simulink model "InverterStartupControl"  (R2022b)
settings: Solver=FixedStepAuto  StartTime=0.0  StopTime=inf  FixedStep=0.005  RelTol=1e-3  EnableMultiTasking=on
undefined symbols (not defined in the file): MI_STATUSES, motor_interface, motor_interface_lib
libraries: simulink x1
settings Model: ExtModeTrigDuration=10  Creator=LinF  LastModifiedBy=LinF
settings SolverCC: AutoInsertRateTranBlk=on
settings OptimizationCC: EnhancedBackFolding=on  PassReuseOutputArgsAs=Individual arguments  ZeroExternalMemoryAtStartup=off  ZeroInternalMemoryAtStartup=off  MaxStackSize=64  OptimizeBlockOrder=speed  DifferentSizesBufferReuse=on  OptimizationCustomize=off  EfficientTunableParamExpr=on
settings DebuggingCC: ParameterTunabilityLossMsg=error
settings HardwareCC: ProdBitPerPointer=32  ProdBitPerSizeT=32  ProdBitPerPtrDiffT=32  ProdLargestAtomicInteger=Long  ProdLargestAtomicFloat=Double  ProdWordSize=32  ProdLongLongMode=on  ProdHWDeviceType=ARM Compatible->ARM Cortex  UseEmbeddedCoderFeatures=off
settings SFSimCC: MATLABDynamicMemAlloc=off
settings RTWCC: Description=Embedded Coder  SystemTargetFile=ert.tlc  HardwareBoard=STM32 Nucleo F767ZI  TLCOptions=-aInlineSetEventsForThisBaseRateFcn=TLC_FALSE -aSuppressMultiTaskScheduler=TLC_FALSE -aRateBasedStepFcn=1  GenCodeOnly=on  TemplateMakefile=ert_default_tmf  Toolchain=GNU Tools for ARM Embedded Processors
settings CodeAppCC: ForceParamTrailComments=on  IgnoreCustomStorageClasses=off  OperatorAnnotations=on  SimulinkDataObjDesc=on  SFDataObjDesc=on  InsertBlockDesc=on
settings ERTTargetCC: SupportNonInlinedSFcns=on  ExtModeTransport=3  ExtModeStaticAlloc=on  ExtModeStaticAllocSize=2000  ExtModeMexFile=ext_xcp  ExtModeIntrfLevel=Level2 - Open

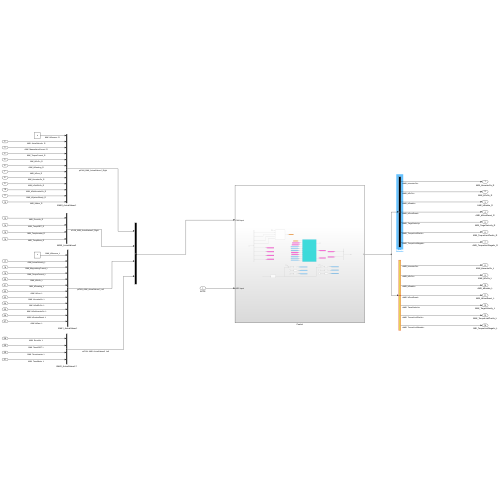
[thumbnail: Simulink's stored preview of the top-level diagram]
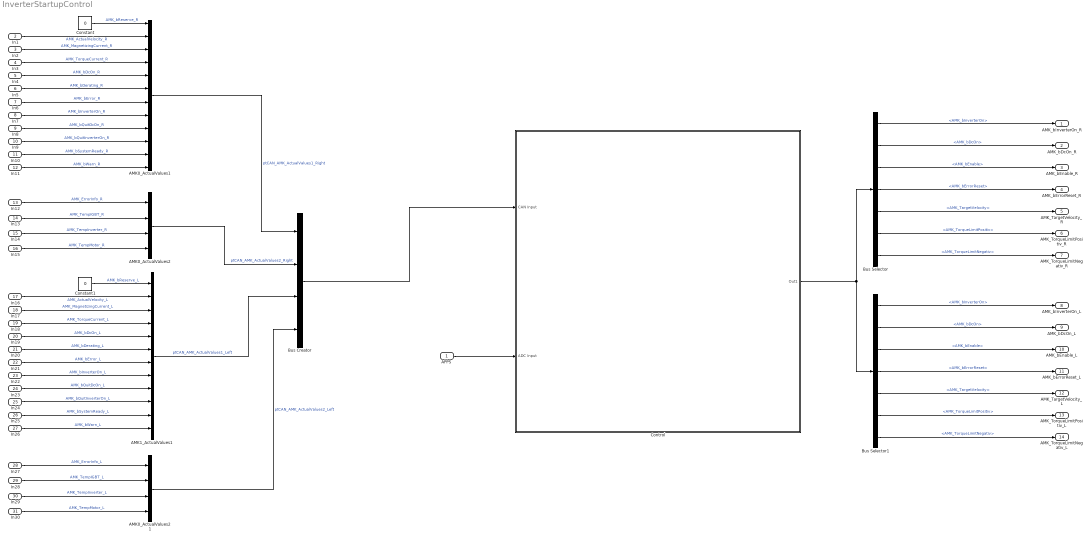
== system InverterStartupControl ==
  APPS : Inport
  In1 : Inport  Port=2
  In2 : Inport  Port=3
  In3 : Inport  Port=4
  In4 : Inport  Port=5
  In5 : Inport  Port=6
  In6 : Inport  Port=7
  In7 : Inport  Port=8
  In8 : Inport  Port=9
  In9 : Inport  Port=10
  In10 : Inport  Port=11
  In11 : Inport  Port=12
  In12 : Inport  Port=13
  In13 : Inport  Port=14
  In14 : Inport  Port=15
  In15 : Inport  Port=16
  In16 : Inport  Port=17
  In17 : Inport  Port=18
  In18 : Inport  Port=19
  In19 : Inport  Port=20
  In20 : Inport  Port=21
  In21 : Inport  Port=22
  In22 : Inport  Port=23
  In23 : Inport  Port=24
  In24 : Inport  Port=25
  In25 : Inport  Port=26
  In26 : Inport  Port=27
  In27 : Inport  Port=28
  In28 : Inport  Port=29
  In29 : Inport  Port=30
  In30 : Inport  Port=31
  "AMK0_ActualValues1 " : BusCreator  Inputs=12
  "AMK0_ActualValues2 " : BusCreator  Inputs=4
  AMK0_ActualValues2 1 : BusCreator  Inputs=4
  AMK1_ActualValues1 : BusCreator  Inputs=12
  Bus Creator : BusCreator  Inputs=4
  Bus Selector : BusSelector  OutputSignals=ptCAN_AMK_Setpoints1_Right.AMK_bInverterOn,ptCAN_AMK_Setpoints1_Right.AMK_bDcOn,ptCAN_AMK_Setpoints1_Right.AMK_bEnable,ptCAN_AMK_Setpoints1_Right.AMK_bErrorReset,ptCAN_AMK_Setpoints1_Right.AMK_TargetVelocity,ptCAN_AMK_Setpoints1_Right.AMK_TorqueLimitPositiv,ptCAN_AMK_Setpoints1_Right.AMK_TorqueLimitNegativ
  Bus Selector1 : BusSelector  OutputSignals=ptCAN_AMK_Setpoints1_Left.AMK_bInverterOn,ptCAN_AMK_Setpoints1_Left.AMK_bDcOn,ptCAN_AMK_Setpoints1_Left.AMK_bEnable,ptCAN_AMK_Setpoints1_Left.AMK_bErrorReset,ptCAN_AMK_Setpoints1_Left.AMK_TargetVelocity,ptCAN_AMK_Setpoints1_Left.AMK_TorqueLimitPositiv,ptCAN_AMK_Setpoints1_Left.AMK_TorqueLimitNegativ
  Constant : Constant  Value=0
  Constant1 : Constant  Value=0
  Control : Subsystem
  AMK_bInverterOn_R : Outport
  AMK_bDcOn_R : Outport  Port=2
  AMK_bEnable_R : Outport  Port=3
  AMK_bErrorReset_R : Outport  Port=4
  AMK_TargetVelocity_R : Outport  Port=5
  AMK_TorqueLimitPositiv_R : Outport  Port=6
  AMK_TorqueLimitNegativ_R : Outport  Port=7
  AMK_bInverterOn_L : Outport  Port=8
  AMK_bDcOn_L : Outport  Port=9
  AMK_bEnable_L : Outport  Port=10
  AMK_bErrorReset_L : Outport  Port=11
  AMK_TargetVelocity_L : Outport  Port=12
  AMK_TorqueLimitPositiv_L : Outport  Port=13
  AMK_TorqueLimitNegativ_L : Outport  Port=14
  wires:
  Bus Selector1/1 -> AMK_bInverterOn_L/1  "<AMK_bInverterOn>"
  Bus Selector/1 -> AMK_bInverterOn_R/1  "<AMK_bInverterOn>"
  Bus Selector1/7 -> AMK_TorqueLimitNegativ_L/1  "<AMK_TorqueLimitNegativ>"
  Bus Selector1/4 -> AMK_bErrorReset_L/1  "<AMK_bErrorReset>"
  Bus Selector1/3 -> AMK_bEnable_L/1  "<AMK_bEnable>"
  Bus Selector/5 -> AMK_TargetVelocity_R/1  "<AMK_TargetVelocity>"
  Bus Selector/4 -> AMK_bErrorReset_R/1  "<AMK_bErrorReset>"
  Bus Selector/3 -> AMK_bEnable_R/1  "<AMK_bEnable>"
  Bus Selector/7 -> AMK_TorqueLimitNegativ_R/1  "<AMK_TorqueLimitNegativ>"
  Bus Selector/6 -> AMK_TorqueLimitPositiv_R/1  "<AMK_TorqueLimitPositiv>"
  Bus Selector1/5 -> AMK_TargetVelocity_L/1  "<AMK_TargetVelocity>"
  Bus Selector1/6 -> AMK_TorqueLimitPositiv_L/1  "<AMK_TorqueLimitPositiv>"
  Bus Selector/2 -> AMK_bDcOn_R/1  "<AMK_bDcOn>"
  Control/1(Out1) -> Bus Selector/1, Bus Selector1/1
  Bus Selector1/2 -> AMK_bDcOn_L/1  "<AMK_bDcOn>"
  APPS/1 -> Control/2(ADC Input)
  In16/1 -> AMK1_ActualValues1/2  "AMK_ActualVelocity_L"
  In21/1 -> AMK1_ActualValues1/7  "AMK_bError_L"
  In11/1 -> "AMK0_ActualValues1 "/12  "AMK_bWarn_R"
  In10/1 -> "AMK0_ActualValues1 "/11  "AMK_bSystemReady_R"
  In28/1 -> AMK0_ActualValues2 1/2  "AMK_TempIGBT_L"
  In18/1 -> AMK1_ActualValues1/4  "AMK_TorqueCurrent_L"
  In4/1 -> "AMK0_ActualValues1 "/5  "AMK_bDcOn_R"
  In9/1 -> "AMK0_ActualValues1 "/10  "AMK_bQuitInverterOn_R"
  In25/1 -> AMK1_ActualValues1/11  "AMK_bSystemReady_L"
  In19/1 -> AMK1_ActualValues1/5  "AMK_bDcOn_L"
  In22/1 -> AMK1_ActualValues1/8  "AMK_bInverterOn_L"
  In12/1 -> "AMK0_ActualValues2 "/1  "AMK_ErrorInfo_R"
  In23/1 -> AMK1_ActualValues1/9  "AMK_bQuitDcOn_L"
  In30/1 -> AMK0_ActualValues2 1/4  "AMK_TempMotor_L"
  In6/1 -> "AMK0_ActualValues1 "/7  "AMK_bError_R"
  In27/1 -> AMK0_ActualValues2 1/1  "AMK_ErrorInfo_L"
  In17/1 -> AMK1_ActualValues1/3  "AMK_MagnetizingCurrent_L"
  In29/1 -> AMK0_ActualValues2 1/3  "AMK_TempInverter_L"
  In1/1 -> "AMK0_ActualValues1 "/2  "AMK_ActualVelocity_R"
  In5/1 -> "AMK0_ActualValues1 "/6  "AMK_bDerating_R"
  In24/1 -> AMK1_ActualValues1/10  "AMK_bQuitInverterOn_L"
  In20/1 -> AMK1_ActualValues1/6  "AMK_bDerating_L"
  In15/1 -> "AMK0_ActualValues2 "/4  "AMK_TempMotor_R"
  In14/1 -> "AMK0_ActualValues2 "/3  "AMK_TempInverter_R"
  AMK1_ActualValues1/1 -> Bus Creator/3  "ptCAN_AMK_ActualValues1_Left"
  In13/1 -> "AMK0_ActualValues2 "/2  "AMK_TempIGBT_R"
  Constant1/1 -> AMK1_ActualValues1/1  "AMK_bReserve_L"
  In8/1 -> "AMK0_ActualValues1 "/9  "AMK_bQuitDcOn_R"
  In3/1 -> "AMK0_ActualValues1 "/4  "AMK_TorqueCurrent_R"
  AMK0_ActualValues2 1/1 -> Bus Creator/4  "ptCAN_AMK_ActualValues2_Left"
  In2/1 -> "AMK0_ActualValues1 "/3  "AMK_MagnetizingCurrent_R"
  Bus Creator/1 -> Control/1(CAN Input)
  Constant/1 -> "AMK0_ActualValues1 "/1  "AMK_bReserve_R"
  "AMK0_ActualValues1 "/1 -> Bus Creator/1  "ptCAN_AMK_ActualValues1_Right"
  In7/1 -> "AMK0_ActualValues1 "/8  "AMK_bInverterOn_R"
  In26/1 -> AMK1_ActualValues1/12  "AMK_bWarn_L"
  "AMK0_ActualValues2 "/1 -> Bus Creator/2  "ptCAN_AMK_ActualValues2_Right"

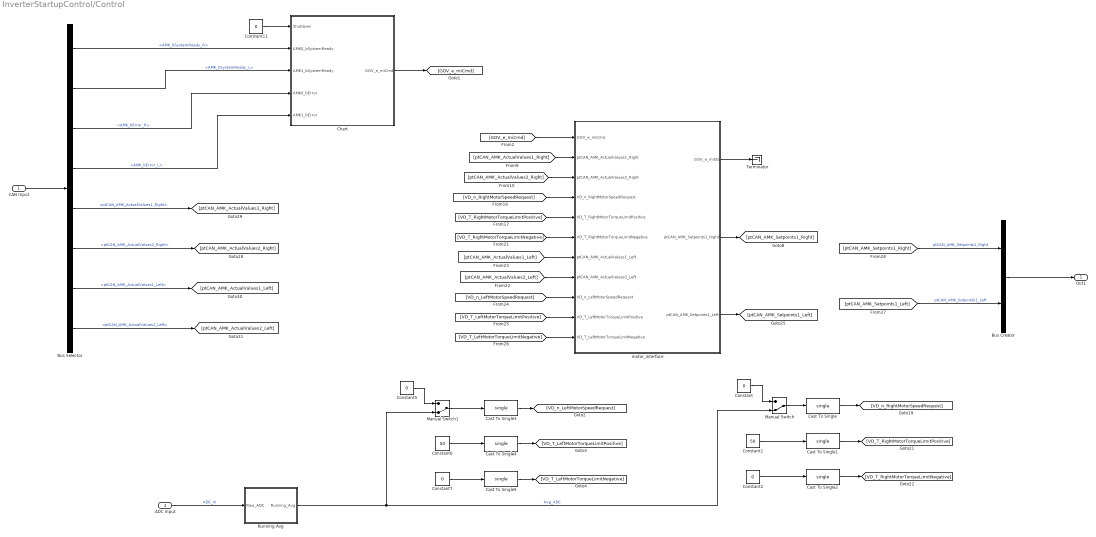
== system InverterStartupControl/Control ==
  CAN Input : Inport
  ADC Input : Inport  Port=2
  Bus Creator : BusCreator  Inputs=2
  Bus Selector : BusSelector  OutputSignals=ptCAN_AMK_ActualValues1_Right.AMK_bSystemReady_R,ptCAN_AMK_ActualValues1_Left.AMK_bSystemReady_L,ptCAN_AMK_ActualValues1_Right.AMK_bError_R,ptCAN_AMK_ActualValues1_Left.AMK_bError_L,ptCAN_AMK_ActualValues1_Right,ptCAN_AMK_ActualValues2_Right,ptCAN_AMK_ActualValues1_Left,ptCAN_AMK_ActualValues2_Left
  Cast To Single{,1..5} (6 alike) : DataTypeConversion  OutDataTypeStr=single  SaturateOnIntegerOverflow=off  RndMeth=Floor
  Chart : Stateflow chart  TreatAsAtomicUnit=on
  Constant{,2,5,7,11} (5 alike) : Constant  Value=0
  Constant1 : Constant  Value=50
  Constant6 : Constant  Value=50
  Manual Switch : ManualSwitch  CurrentSetting=0
  Manual Switch1 : ManualSwitch  CurrentSetting=0
  Running Avg : Subsystem
  Terminator : Terminator
  motor_interface : Subsystem  AncestorBlock=motor_interface_lib/motor_interface
      settings: LibrarySourceBlock=motor_interface_lib/motor_interface
  Out1 : Outport
  wires:
  [VD_T_RightMotorTorqueLimitPositive] -> motor_interface/5(VD_T_RightMotorTorqueLimitPositive)
  [ptCAN_AMK_ActualValues2_Right] -> motor_interface/3(ptCAN_AMK_ActualValues2_Right)
  [ptCAN_AMK_ActualValues2_Left] -> motor_interface/8(ptCAN_AMK_ActualValues2_Left)
  [VD_n_LeftMotorSpeedRequest] -> motor_interface/9(VD_n_LeftMotorSpeedRequest)
  [VD_T_LeftMotorTorqueLimitNegative] -> motor_interface/11(VD_T_LeftMotorTorqueLimitNegative)
  [VD_T_RightMotorTorqueLimitNegative] -> motor_interface/6(VD_T_RightMotorTorqueLimitNegative)
  motor_interface/2(ptCAN_AMK_Setpoints1_Right) -> [ptCAN_AMK_Setpoints1_Right]
  motor_interface/3(ptCAN_AMK_Setpoints1_Left) -> [ptCAN_AMK_Setpoints1_Left]
  [VD_T_LeftMotorTorqueLimitPositive] -> motor_interface/10(VD_T_LeftMotorTorqueLimitPositive)
  [VD_n_RightMotorSpeedRequest] -> motor_interface/4(VD_n_RightMotorSpeedRequest)
  [ptCAN_AMK_ActualValues1_Left] -> motor_interface/7(ptCAN_AMK_ActualValues1_Left)
  motor_interface/1(GOV_e_miSts) -> Terminator/1
  [GOV_e_miCmd] -> motor_interface/1(GOV_e_miCmd)
  [ptCAN_AMK_ActualValues1_Right] -> motor_interface/2(ptCAN_AMK_ActualValues1_Right)
  CAN Input/1 -> Bus Selector/1
  Bus Selector/6 -> [ptCAN_AMK_ActualValues2_Right]  "<ptCAN_AMK_ActualValues2_Right>"
  Constant2/1 -> Cast To Single2/1
  Bus Selector/8 -> [ptCAN_AMK_ActualValues2_Left]  "<ptCAN_AMK_ActualValues2_Left>"
  Constant7/1 -> Cast To Single5/1
  Manual Switch1/1 -> Cast To Single3/1
  Chart/1(GOV_e_miCmd) -> [GOV_e_miCmd]
  [ptCAN_AMK_Setpoints1_Right] -> Bus Creator/1  "ptCAN_AMK_Setpoints1_Right"
  [ptCAN_AMK_Setpoints1_Left] -> Bus Creator/2  "ptCAN_AMK_Setpoints1_Left"
  Bus Creator/1 -> Out1/1
  Bus Selector/5 -> [ptCAN_AMK_ActualValues1_Right]  "<ptCAN_AMK_ActualValues1_Right>"
  Bus Selector/1 -> Chart/2(AMK0_bSystemReady)  "<AMK_bSystemReady_R>"
  Bus Selector/3 -> Chart/4(AMK0_bError)  "<AMK_bError_R>"
  Constant/1 -> Manual Switch/1
  Manual Switch/1 -> Cast To Single/1
  Constant11/1 -> Chart/1(Shutdown)
  Bus Selector/7 -> [ptCAN_AMK_ActualValues1_Left]  "<ptCAN_AMK_ActualValues1_Left>"
  Cast To Single/1 -> [VD_n_RightMotorSpeedRequest]
  Cast To Single1/1 -> [VD_T_RightMotorTorqueLimitPositive]
  Cast To Single2/1 -> [VD_T_RightMotorTorqueLimitNegative]
  Cast To Single3/1 -> [VD_n_LeftMotorSpeedRequest]
  Cast To Single4/1 -> [VD_T_LeftMotorTorqueLimitPositive]
  Cast To Single5/1 -> [VD_T_LeftMotorTorqueLimitNegative]
  Bus Selector/2 -> Chart/3(AMK1_bSystemReady)  "<AMK_bSystemReady_L>"
  Bus Selector/4 -> Chart/5(AMK1_bError)  "<AMK_bError_L>"
  Constant5/1 -> Manual Switch1/1
  ADC Input/1 -> Running Avg/1(Raw_ADC)  "ADC_In"
  Running Avg/1(Running_Avg) -> Manual Switch/2, Manual Switch1/2  "Avg_ADC"
  Constant1/1 -> Cast To Single1/1
  Constant6/1 -> Cast To Single4/1

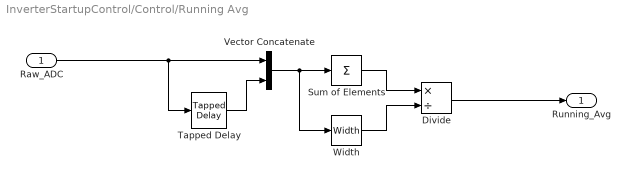
== system InverterStartupControl/Control/Running Avg ==
  Raw_ADC : Inport
  Divide : Product  Inputs=*/
  Sum of Elements : Sum  Inputs=+
  Tapped Delay : simulink/Discrete/Tapped Delay  vinit=0  samptime=-1  NumDelays=5  DelayOrder=Oldest  includeCurrent=off
  Vector Concatenate : Concatenate
  Width : Width
  Running_Avg : Outport
  wires:
  Divide/1 -> Running_Avg/1
  Vector Concatenate/1 -> Width/1, Sum of Elements/1
  Raw_ADC/1 -> Vector Concatenate/1, Tapped Delay/1
  Width/1 -> Divide/2
  Tapped Delay/1 -> Vector Concatenate/2
  Sum of Elements/1 -> Divide/1

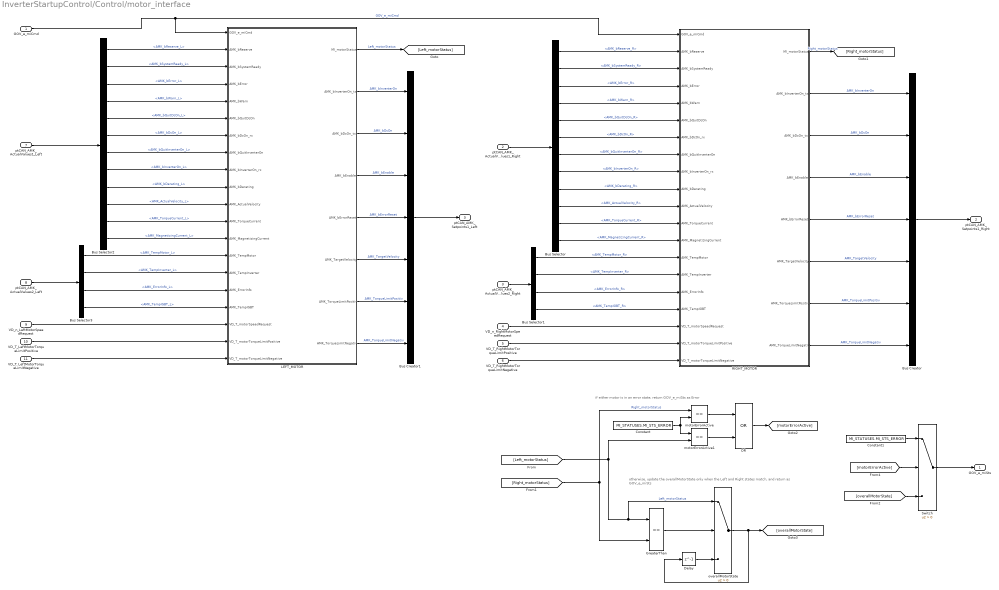
== system InverterStartupControl/Control/motor_interface ==
  note: otherwise, update the overallMotorState only when the Left and Right states match, and return as GOV_e_miSts
  note: if either motor is in an error state, return GOV_e_miSts as Error
  GOV_e_miCmd : Inport
  ptCAN_AMK_ActualValues1_Right : Inport  Port=2
  ptCAN_AMK_ActualValues2_Right : Inport  Port=3
  VD_n_RightMotorSpeedRequest : Inport  Port=4
  VD_T_RightMotorTorqueLimitPositive : Inport  Port=5
  VD_T_RightMotorTorqueLimitNegative : Inport  Port=6
  ptCAN_AMK_ActualValues1_Left : Inport  Port=7
  ptCAN_AMK_ActualValues2_Left : Inport  Port=8
  VD_n_LeftMotorSpeedRequest : Inport  Port=9
  VD_T_LeftMotorTorqueLimitPositive : Inport  Port=10
  VD_T_LeftMotorTorqueLimitNegative : Inport  Port=11
  Bus Creator : BusCreator  Inputs=7
  Bus Creator1 : BusCreator  Inputs=7
  Bus Selector : BusSelector  OutputSignals=AMK_bReserve_R,AMK_bSystemReady_R,AMK_bError_R,AMK_bWarn_R,AMK_bQuitDcOn_R,AMK_bDcOn_R,AMK_bQuitInverterOn_R,AMK_bInverterOn_R,AMK_bDerating_R,AMK_ActualVelocity_R,AMK_TorqueCurrent_R,AMK_MagnetizingCurrent_R
  Bus Selector1 : BusSelector  OutputSignals=AMK_TempMotor_R,AMK_TempInverter_R,AMK_ErrorInfo_R,AMK_TempIGBT_R
  Bus Selector2 : BusSelector  OutputSignals=AMK_bReserve_L,AMK_bSystemReady_L,AMK_bError_L,AMK_bWarn_L,AMK_bQuitDcOn_L,AMK_bDcOn_L,AMK_bQuitInverterOn_L,AMK_bInverterOn_L,AMK_bDerating_L,AMK_ActualVelocity_L,AMK_TorqueCurrent_L,AMK_MagnetizingCurrent_L
  Bus Selector3 : BusSelector  OutputSignals=AMK_TempMotor_L,AMK_TempInverter_L,AMK_ErrorInfo_L,AMK_TempIGBT_L
  Constant : Constant  Value=MI_STATUSES.MI_STS_ERROR  OutDataTypeStr=Enum: MI_STATUSES
  Constant1 : Constant  Value=MI_STATUSES.MI_STS_ERROR  OutDataTypeStr=Enum: MI_STATUSES
  Delay : Delay  DelayLength=1  InitialCondition=MI_STATUSES.OFF
  GreaterThan : RelationalOperator  Operator===  OutDataTypeStr=boolean  RndMeth=Simplest  InputSameDT=off
  LEFT_MOTOR : Stateflow chart  TreatAsAtomicUnit=on
  OR : Logic  Operator=OR  IconShape=distinctive  AllPortsSameDT=off  OutDataTypeStr=boolean
  RIGHT_MOTOR : Stateflow chart  TreatAsAtomicUnit=on
  Switch : Switch  Criteria=u2 > Threshold  SaturateOnIntegerOverflow=off  InputSameDT=off
  motorErrorActive : RelationalOperator  Operator===  OutDataTypeStr=boolean  RndMeth=Simplest  InputSameDT=off
  motorErrorActive1 : RelationalOperator  Operator===  OutDataTypeStr=boolean  RndMeth=Simplest  InputSameDT=off
  overallMotorState : Switch  Criteria=u2 > Threshold  SaturateOnIntegerOverflow=off  InputSameDT=off
  GOV_e_miSts : Outport
  ptCAN_AMK_Setpoints1_Right : Outport  Port=2
  ptCAN_AMK_Setpoints1_Left : Outport  Port=3
  wires:
  GOV_e_miCmd/1 -> LEFT_MOTOR/1(GOV_e_miCmd), RIGHT_MOTOR/1(GOV_e_miCmd)  "GOV_e_miCmd"
  ptCAN_AMK_ActualValues1_Right/1 -> Bus Selector/1
  Bus Selector/2 -> RIGHT_MOTOR/3(AMK_bSystemReady)  "<AMK_bSystemReady_R>"
  Bus Selector/3 -> RIGHT_MOTOR/4(AMK_bError)  "<AMK_bError_R>"
  Bus Selector/4 -> RIGHT_MOTOR/5(AMK_bWarn)  "<AMK_bWarn_R>"
  Bus Selector/5 -> RIGHT_MOTOR/6(AMK_bQuitDcOn)  "<AMK_bQuitDcOn_R>"
  Bus Selector/6 -> RIGHT_MOTOR/7(AMK_bDcOn_rx)  "<AMK_bDcOn_R>"
  Bus Selector/7 -> RIGHT_MOTOR/8(AMK_bQuitInverterOn)  "<AMK_bQuitInverterOn_R>"
  Bus Selector/8 -> RIGHT_MOTOR/9(AMK_bInverterOn_rx)  "<AMK_bInverterOn_R>"
  Bus Selector/9 -> RIGHT_MOTOR/10(AMK_bDerating)  "<AMK_bDerating_R>"
  Bus Selector/10 -> RIGHT_MOTOR/11(AMK_ActualVelocity)  "<AMK_ActualVelocity_R>"
  Bus Selector/11 -> RIGHT_MOTOR/12(AMK_TorqueCurrent)  "<AMK_TorqueCurrent_R>"
  Bus Selector/12 -> RIGHT_MOTOR/13(AMK_MagnetizingCurrent)  "<AMK_MagnetizingCurrent_R>"
  Bus Selector/1 -> RIGHT_MOTOR/2(AMK_bReserve)  "<AMK_bReserve_R>"
  ptCAN_AMK_ActualValues2_Right/1 -> Bus Selector1/1
  Bus Selector1/1 -> RIGHT_MOTOR/14(AMK_TempMotor)  "<AMK_TempMotor_R>"
  Bus Selector1/2 -> RIGHT_MOTOR/15(AMK_TempInverter)  "<AMK_TempInverter_R>"
  Bus Selector1/3 -> RIGHT_MOTOR/16(AMK_ErrorInfo)  "<AMK_ErrorInfo_R>"
  Bus Selector1/4 -> RIGHT_MOTOR/17(AMK_TempIGBT)  "<AMK_TempIGBT_R>"
  Bus Creator/1 -> ptCAN_AMK_Setpoints1_Right/1
  RIGHT_MOTOR/2(AMK_bInverterOn_tx) -> Bus Creator/1  "AMK_bInverterOn"
  RIGHT_MOTOR/4(AMK_bEnable) -> Bus Creator/3  "AMK_bEnable"
  RIGHT_MOTOR/6(AMK_TargetVelocity) -> Bus Creator/5  "AMK_TargetVelocity"
  RIGHT_MOTOR/3(AMK_bDcOn_tx) -> Bus Creator/2  "AMK_bDcOn"
  RIGHT_MOTOR/5(AMK_bErrorReset) -> Bus Creator/4  "AMK_bErrorReset"
  LEFT_MOTOR/1(MI_motorStatus) -> [Left_motorStatus]  "Left_motorStatus"
  RIGHT_MOTOR/1(MI_motorStatus) -> [Right_motorStatus]  "Right_motorStatus"
  [Left_motorStatus] -> motorErrorActive1/2, overallMotorState/1, GreaterThan/1  "Left_motorStatus"
  [Right_motorStatus] -> motorErrorActive/1, GreaterThan/2  "Right_motorStatus"
  Constant/1 -> motorErrorActive/2, motorErrorActive1/1
  Switch/1 -> GOV_e_miSts/1
  [motorErrorActive] -> Switch/2
  overallMotorState/1 -> Delay/1, [overallMotorState]
  Delay/1 -> overallMotorState/3
  GreaterThan/1 -> overallMotorState/2
  [overallMotorState] -> Switch/3
  OR/1 -> [motorErrorActive]
  motorErrorActive1/1 -> OR/2
  motorErrorActive/1 -> OR/1
  Constant1/1 -> Switch/1
  RIGHT_MOTOR/7(AMK_TorqueLimitPositiv) -> Bus Creator/6  "AMK_TorqueLimitPositiv"
  RIGHT_MOTOR/8(AMK_TorqueLimitNegativ) -> Bus Creator/7  "AMK_TorqueLimitNegativ"
  VD_T_RightMotorTorqueLimitPositive/1 -> RIGHT_MOTOR/19(VD_T_motorTorqueLimitPositive)
  VD_T_RightMotorTorqueLimitNegative/1 -> RIGHT_MOTOR/20(VD_T_motorTorqueLimitNegative)
  VD_n_RightMotorSpeedRequest/1 -> RIGHT_MOTOR/18(VD_T_motorSpeedRequest)
  VD_n_LeftMotorSpeedRequest/1 -> LEFT_MOTOR/18(VD_T_motorSpeedRequest)
  VD_T_LeftMotorTorqueLimitNegative/1 -> LEFT_MOTOR/20(VD_T_motorTorqueLimitNegative)
  VD_T_LeftMotorTorqueLimitPositive/1 -> LEFT_MOTOR/19(VD_T_motorTorqueLimitPositive)
  Bus Selector3/4 -> LEFT_MOTOR/17(AMK_TempIGBT)  "<AMK_TempIGBT_L>"
  Bus Selector3/3 -> LEFT_MOTOR/16(AMK_ErrorInfo)  "<AMK_ErrorInfo_L>"
  Bus Selector3/2 -> LEFT_MOTOR/15(AMK_TempInverter)  "<AMK_TempInverter_L>"
  Bus Selector3/1 -> LEFT_MOTOR/14(AMK_TempMotor)  "<AMK_TempMotor_L>"
  Bus Selector2/1 -> LEFT_MOTOR/2(AMK_bReserve)  "<AMK_bReserve_L>"
  Bus Selector2/12 -> LEFT_MOTOR/13(AMK_MagnetizingCurrent)  "<AMK_MagnetizingCurrent_L>"
  Bus Selector2/11 -> LEFT_MOTOR/12(AMK_TorqueCurrent)  "<AMK_TorqueCurrent_L>"
  Bus Selector2/10 -> LEFT_MOTOR/11(AMK_ActualVelocity)  "<AMK_ActualVelocity_L>"
  Bus Selector2/9 -> LEFT_MOTOR/10(AMK_bDerating)  "<AMK_bDerating_L>"
  Bus Selector2/8 -> LEFT_MOTOR/9(AMK_bInverterOn_rx)  "<AMK_bInverterOn_L>"
  Bus Selector2/7 -> LEFT_MOTOR/8(AMK_bQuitInverterOn)  "<AMK_bQuitInverterOn_L>"
  Bus Selector2/6 -> LEFT_MOTOR/7(AMK_bDcOn_rx)  "<AMK_bDcOn_L>"
  Bus Selector2/5 -> LEFT_MOTOR/6(AMK_bQuitDcOn)  "<AMK_bQuitDcOn_L>"
  Bus Selector2/4 -> LEFT_MOTOR/5(AMK_bWarn)  "<AMK_bWarn_L>"
  Bus Selector2/3 -> LEFT_MOTOR/4(AMK_bError)  "<AMK_bError_L>"
  Bus Selector2/2 -> LEFT_MOTOR/3(AMK_bSystemReady)  "<AMK_bSystemReady_L>"
  ptCAN_AMK_ActualValues1_Left/1 -> Bus Selector2/1
  LEFT_MOTOR/8(AMK_TorqueLimitNegativ) -> Bus Creator1/7  "AMK_TorqueLimitNegativ"
  LEFT_MOTOR/7(AMK_TorqueLimitPositiv) -> Bus Creator1/6  "AMK_TorqueLimitPositiv"
  LEFT_MOTOR/5(AMK_bErrorReset) -> Bus Creator1/4  "AMK_bErrorReset"
  LEFT_MOTOR/3(AMK_bDcOn_tx) -> Bus Creator1/2  "AMK_bDcOn"
  LEFT_MOTOR/6(AMK_TargetVelocity) -> Bus Creator1/5  "AMK_TargetVelocity"
  LEFT_MOTOR/4(AMK_bEnable) -> Bus Creator1/3  "AMK_bEnable"
  LEFT_MOTOR/2(AMK_bInverterOn_tx) -> Bus Creator1/1  "AMK_bInverterOn"
  Bus Creator1/1 -> ptCAN_AMK_Setpoints1_Left/1
  ptCAN_AMK_ActualValues2_Left/1 -> Bus Selector3/1

== stateflow chart InverterStartupControl/Control/Chart ==
  state Init
    en:
    GOV_e_miCmd = MI_CMD.CMD_INIT;
  state Run
    en:
    GOV_e_miCmd = MI_CMD.CMD_STARTUP;
  state Error0
    en:
    GOV_e_miCmd = MI_CMD.ERR_RESET;
  state Error1
    en:
    GOV_e_miCmd = MI_CMD.ERR_RESET;
  state Shutdown
    en:
    GOV_e_miCmd = MI_CMD.CMD_SHUTDOWN;
  (default) -> Init
  Shutdown -> Init : [Shutdown == 0]
  Init -> Run : [(AMK0_bSystemReady == 1 && AMK1_bSystemReady == 1) && Shutdown == 0]
  Run -> Error0 [order 1] : [AMK0_bError == 1]
  Error0 -> Run : [AMK0_bError == 0]
  Run -> Error1 [order 3] : [AMK1_bError == 1]
  Error1 -> Run : [AMK1_bError == 0]
  Run -> Shutdown [order 2] : [Shutdown == 1]
  data: Shutdown input; GOV_e_miCmd output; AMK0_bSystemReady input; AMK1_bSystemReady input; AMK0_bError input; AMK1_bError input

== stateflow chart InverterStartupControl/Control/motor_interface/LEFT_MOTOR ==
  note: [AMK_bError==1]
  state motorOff_waitingForGov
    en:
    MI_motorStatus = MI_STATUSES.OFF;
    AMK_bInverterOn_tx = 0;
    AMK_bDcOn_tx = 0;
    AMK_bEnable = 0;
    AMK_bErrorReset = 0;
    AMK_TargetVelocity = 0;
    AMK_TorqueLimitPositiv = 0;
    AMK_TorqueLimitNegativ = 0;
  state AMK_startup
    state waiting_sysReady
      en:
      MI_motorStatus = MI_STATUSES.STARTUP;
    state toggleDCon
      en:
      AMK_bDcOn_tx = 1;
    state enforceSetpointsZero
      en:
      AMK_TargetVelocity = 0;
      AMK_TorqueLimitPositiv = 0;
      AMK_TorqueLimitNegativ = 0;
    state commandOn
      en:
      AMK_bEnable = 1;
      AMK_bInverterOn_tx = 1;
    waiting_sysReady -> (junction 67) [order 2] : [AMK_bError==1]
    waiting_sysReady -> AMK_startup.toggleDCon [order 1] : [AMK_bSystemReady==1]
    AMK_startup.toggleDCon -> (junction 67) [order 2] : [AMK_bError==1]
    AMK_startup.toggleDCon -> AMK_startup.enforceSetpointsZero [order 1] : [(AMK_bDcOn_rx==1) ...
        | && (AMK_bQuitDcOn==1)]
    AMK_startup.enforceSetpointsZero -> (junction 67) [order 2] : [AMK_bError==1]
    commandOn -> (junction 67) [order 2] : [AMK_bError==1]
    AMK_startup.enforceSetpointsZero -> commandOn [order 1] : after(1,sec)
  state AMK_errorReset
    state toggleReset
      en:
      AMK_bErrorReset = 0;
    state sendReset
      en:
      AMK_bErrorReset = 1;
    state toggleEnable
      en:
      AMK_bEnable = 0;
    state enforceSetpointsZero
      en:
      AMK_TargetVelocity = 0;
      AMK_TorqueLimitPositiv = 0;
      AMK_TorqueLimitNegativ = 0;
      AMK_bInverterOn_tx = 0;
    sendReset -> toggleReset : after(500,msec)
    toggleEnable -> sendReset : after(500,msec)
    AMK_errorReset.enforceSetpointsZero -> toggleEnable : [AMK_bInverterOn_rx==0]
  state AMK_shutdown
    state toggleDCon
      en:
      AMK_bDcOn_tx = 0;
    state commandOff
      en:
      AMK_bEnable = 0;
    state enforceSetpointsZero
      en:
      MI_motorStatus = MI_STATUSES.SHUTDOWN;
      AMK_TargetVelocity = 0;
      AMK_TorqueLimitPositiv = 0;
      AMK_TorqueLimitNegativ = 0;
      AMK_bInverterOn_tx = 0;
    AMK_shutdown.toggleDCon -> (junction 94) [order 2] : [AMK_bError==1]
    commandOff -> AMK_shutdown.toggleDCon [order 1] : [AMK_bQuitInverterOn==0]
    commandOff -> (junction 94) [order 2] : [AMK_bError==1]
    AMK_shutdown.enforceSetpointsZero -> (junction 94) [order 2] : [AMK_bError==1]
    AMK_shutdown.enforceSetpointsZero -> commandOff [order 1] : [AMK_bInverterOn_rx==0]
  state AMK_errorDetected
    en:
    MI_motorStatus = MI_STATUSES.MI_STS_ERROR;
  state AMK_running
    during:
    MI_motorStatus = MI_STATUSES.RUNNING;
    AMK_TargetVelocity = VD_T_motorSpeedRequest;
    AMK_TorqueLimitPositiv = VD_T_motorTorqueLimitPositive;
    AMK_TorqueLimitNegativ = VD_T_motorTorqueLimitNegative;
  toggleReset -> motorOff_waitingForGov : [AMK_bSystemReady==1]
  AMK_running -> AMK_shutdown.enforceSetpointsZero [order 2] : [GOV_e_miCmd == MI_CMD.CMD_SHUTDOWN]
  commandOn -> AMK_running [order 1] : [(AMK_bInverterOn_rx ==1) && ...
      |  (AMK_bQuitInverterOn==1)]
  AMK_shutdown.toggleDCon -> motorOff_waitingForGov [order 1] : [(AMK_bDcOn_rx==0) && (AMK_bQuitDcOn==0)]
  motorOff_waitingForGov -> waiting_sysReady : [GOV_e_miCmd == MI_CMD.CMD_STARTUP]
  (default) -> motorOff_waitingForGov
  (junction 67) -> AMK_errorDetected
  (junction 94) -> AMK_errorDetected
  AMK_errorDetected -> AMK_errorReset.enforceSetpointsZero : [GOV_e_miCmd == MI_CMD.ERR_RESET]
  AMK_running -> AMK_errorDetected [order 1] : [AMK_bError==1]
  data: GOV_e_miCmd input Enum: MI_CMD; MI_motorStatus output Enum: MI_STATUSES size=1; AMK_bReserve input; AMK_bSystemReady input; AMK_bError input; AMK_bWarn input; AMK_bQuitDcOn input; AMK_bDcOn_rx input; AMK_bQuitInverterOn input; AMK_bInverterOn_rx input; AMK_bDerating input; AMK_ActualVelocity input; AMK_TorqueCurrent input; AMK_MagnetizingCurrent input; AMK_TempMotor input; AMK_TempInverter input; AMK_ErrorInfo input; AMK_TempIGBT input; VD_T_motorSpeedRequest input; AMK_bInverterOn_tx output uint8 size=1; AMK_bDcOn_tx output uint8 size=1; AMK_bEnable output uint8 size=1; AMK_bErrorReset output uint8 size=1; AMK_TargetVelocity output single size=1; AMK_TorqueLimitPositiv output single size=1; AMK_TorqueLimitNegativ output single size=1; VD_T_motorTorqueLimitPositive input; VD_T_motorTorqueLimitNegative input

== stateflow chart InverterStartupControl/Control/motor_interface/RIGHT_MOTOR ==
  note: [AMK_bError==1]
  state motorOff_waitingForGov
    en:
    MI_motorStatus = MI_STATUSES.OFF;
    AMK_bInverterOn_tx = 0;
    AMK_bDcOn_tx = 0;
    AMK_bEnable = 0;
    AMK_bErrorReset = 0;
    AMK_TargetVelocity = 0;
    AMK_TorqueLimitPositiv = 0;
    AMK_TorqueLimitNegativ = 0;
  state AMK_startup
    state waiting_sysReady
      en:
      MI_motorStatus = MI_STATUSES.STARTUP;
    state toggleDCon
      en:
      AMK_bDcOn_tx = 1;
    state enforceSetpointsZero
      en:
      AMK_TargetVelocity = 0;
      AMK_TorqueLimitPositiv = 0;
      AMK_TorqueLimitNegativ = 0;
    state commandOn
      en:
      AMK_bEnable = 1;
      AMK_bInverterOn_tx = 1;
    waiting_sysReady -> (junction 67) [order 2] : [AMK_bError==1]
    waiting_sysReady -> AMK_startup.toggleDCon [order 1] : [AMK_bSystemReady==1]
    AMK_startup.toggleDCon -> (junction 67) [order 2] : [AMK_bError==1]
    AMK_startup.toggleDCon -> AMK_startup.enforceSetpointsZero [order 1] : [(AMK_bDcOn_rx==1) ...
        | && (AMK_bQuitDcOn==1)]
    AMK_startup.enforceSetpointsZero -> (junction 67) [order 2] : [AMK_bError==1]
    commandOn -> (junction 67) [order 2] : [AMK_bError==1]
    AMK_startup.enforceSetpointsZero -> commandOn [order 1] : after(1,sec)
  state AMK_errorReset
    state toggleReset
      en:
      AMK_bErrorReset = 0;
    state sendReset
      en:
      AMK_bErrorReset = 1;
    state toggleEnable
      en:
      AMK_bEnable = 0;
    state enforceSetpointsZero
      en:
      AMK_TargetVelocity = 0;
      AMK_TorqueLimitPositiv = 0;
      AMK_TorqueLimitNegativ = 0;
      AMK_bInverterOn_tx = 0;
    sendReset -> toggleReset : after(500,msec)
    toggleEnable -> sendReset : after(500,msec)
    AMK_errorReset.enforceSetpointsZero -> toggleEnable : [AMK_bInverterOn_rx==0]
  state AMK_shutdown
    state toggleDCon
      en:
      AMK_bDcOn_tx = 0;
    state commandOff
      en:
      AMK_bEnable = 0;
    state enforceSetpointsZero
      en:
      MI_motorStatus = MI_STATUSES.SHUTDOWN;
      AMK_TargetVelocity = 0;
      AMK_TorqueLimitPositiv = 0;
      AMK_TorqueLimitNegativ = 0;
      AMK_bInverterOn_tx = 0;
    AMK_shutdown.toggleDCon -> (junction 94) [order 2] : [AMK_bError==1]
    commandOff -> AMK_shutdown.toggleDCon [order 1] : [AMK_bQuitInverterOn==0]
    commandOff -> (junction 94) [order 2] : [AMK_bError==1]
    AMK_shutdown.enforceSetpointsZero -> (junction 94) [order 2] : [AMK_bError==1]
    AMK_shutdown.enforceSetpointsZero -> commandOff [order 1] : [AMK_bInverterOn_rx==0]
  state AMK_errorDetected
    en:
    MI_motorStatus = MI_STATUSES.MI_STS_ERROR;
  state AMK_running
    during:
    MI_motorStatus = MI_STATUSES.RUNNING;
    AMK_TargetVelocity = VD_T_motorSpeedRequest;
    AMK_TorqueLimitPositiv = VD_T_motorTorqueLimitPositive;
    AMK_TorqueLimitNegativ = VD_T_motorTorqueLimitNegative;
  toggleReset -> motorOff_waitingForGov : [AMK_bSystemReady==1]
  AMK_running -> AMK_shutdown.enforceSetpointsZero [order 2] : [GOV_e_miCmd == MI_CMD.CMD_SHUTDOWN]
  commandOn -> AMK_running [order 1] : [(AMK_bInverterOn_rx ==1) && ...
      |  (AMK_bQuitInverterOn==1)]
  AMK_shutdown.toggleDCon -> motorOff_waitingForGov [order 1] : [(AMK_bDcOn_rx==0) && (AMK_bQuitDcOn==0)]
  motorOff_waitingForGov -> waiting_sysReady : [GOV_e_miCmd == MI_CMD.CMD_STARTUP]
  (default) -> motorOff_waitingForGov
  (junction 67) -> AMK_errorDetected
  (junction 94) -> AMK_errorDetected
  AMK_errorDetected -> AMK_errorReset.enforceSetpointsZero : [GOV_e_miCmd == MI_CMD.ERR_RESET]
  AMK_running -> AMK_errorDetected [order 1] : [AMK_bError==1]
  data: GOV_e_miCmd input Enum: MI_CMD; MI_motorStatus output Enum: MI_STATUSES size=1; AMK_bReserve input; AMK_bSystemReady input; AMK_bError input; AMK_bWarn input; AMK_bQuitDcOn input; AMK_bDcOn_rx input; AMK_bQuitInverterOn input; AMK_bInverterOn_rx input; AMK_bDerating input; AMK_ActualVelocity input; AMK_TorqueCurrent input; AMK_MagnetizingCurrent input; AMK_TempMotor input; AMK_TempInverter input; AMK_ErrorInfo input; AMK_TempIGBT input; VD_T_motorSpeedRequest input; AMK_bInverterOn_tx output uint8 size=1; AMK_bDcOn_tx output uint8 size=1; AMK_bEnable output uint8 size=1; AMK_bErrorReset output uint8 size=1; AMK_TargetVelocity output single size=1; AMK_TorqueLimitPositiv output single size=1; AMK_TorqueLimitNegativ output single size=1; VD_T_motorTorqueLimitPositive input; VD_T_motorTorqueLimitNegative input
